simulink model "Part4_solarpanel"  (R2022b)
settings: Solver=FixedStepAuto  StartTime=0.0  StopTime=20  FixedStep=0.0001  RelTol=1e-3
libraries: fl_lib x8, nesl_utility x8, ee_lib x2, simulink x2
settings Model: Creator=mingreico  LastModifiedBy=mingreico

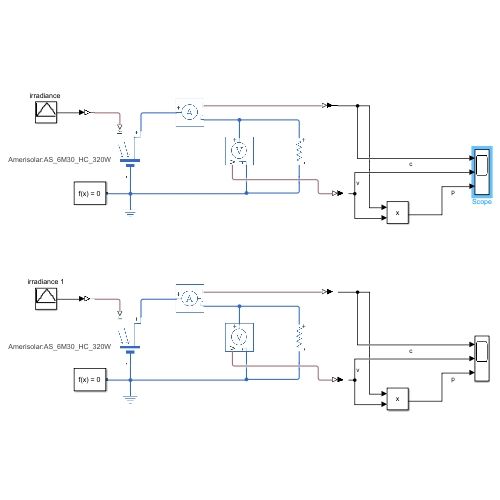
[thumbnail: Simulink's stored preview of the top-level diagram]
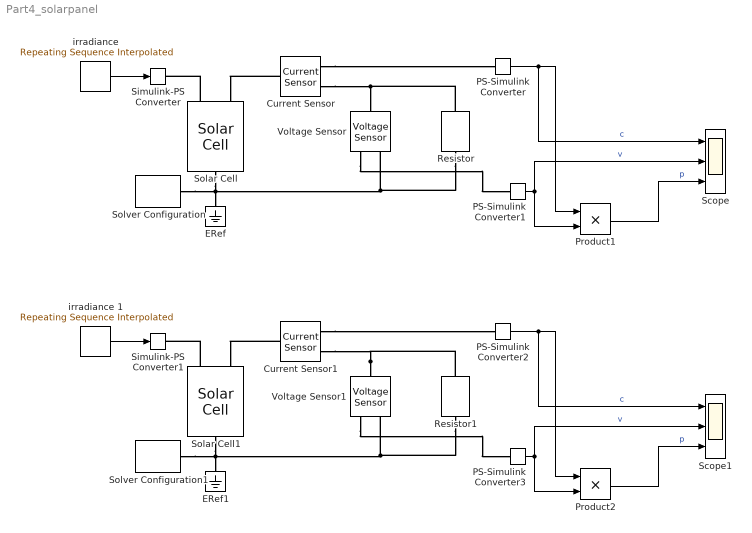
== system Part4_solarpanel ==
  Current Sensor : fl_lib/Electrical/Electrical Sensors/Current Sensor
  Current Sensor1 : fl_lib/Electrical/Electrical Sensors/Current Sensor
  ERef : fl_lib/Electrical/Electrical Elements/Electrical Reference
  ERef1 : fl_lib/Electrical/Electrical Elements/Electrical Reference
  PS-Simulink Converter{,1..3} (4 alike) : nesl_utility/PS-Simulink Converter  PhysicalDomain=network_engine_domain  SubClassName=ps_output  LeftPortType=input  RightPortType=output  PseudoPeriodic=off  Frequencies=[]  VectorFormat=inherit  Unit=inherit  AffineConversion=off
  Product1 : Product
  Product2 : Product
  Resistor : fl_lib/Electrical/Electrical Elements/Resistor  R=100 Ohm  i_specify=off  i_priority=None  i=0 A  i_nominal_specify=off  i_nominal_unit=A  i_nominal_value=1  v_specify=off  v_priority=None  v=0 V  v_nominal_specify=off  v_nominal_unit=V  v_nominal_value=1
  Resistor1 : fl_lib/Electrical/Electrical Elements/Resistor  R=100 Ohm  i_specify=off  i_priority=None  i=0 A  i_nominal_specify=off  i_nominal_unit=A  i_nominal_value=1  v_specify=off  v_priority=None  v=0 V  v_nominal_specify=off  v_nominal_unit=V  v_nominal_value=1
  Scope : Scope  NumInputPorts=3
  Scope1 : Scope  NumInputPorts=3
  Simulink-PS Converter : nesl_utility/Simulink-PS Converter  PhysicalDomain=network_engine_domain  SubClassName=ps_input  LeftPortType=input  RightPortType=output  PseudoPeriodic=off  Frequencies=[]  NoiseDistribution=none  NoiseParameters=[]  Unit=1  AffineConversion=off  FilteringAndDerivatives=provide  SimscapeFilterOrder=1  InputFilterTimeConstant=0.001  UdotUserProvided=0
  Simulink-PS Converter1 : nesl_utility/Simulink-PS Converter  PhysicalDomain=network_engine_domain  SubClassName=ps_input  LeftPortType=input  RightPortType=output  PseudoPeriodic=off  Frequencies=[]  NoiseDistribution=none  NoiseParameters=[]  Unit=1  AffineConversion=off  FilteringAndDerivatives=provide  SimscapeFilterOrder=1  InputFilterTimeConstant=0.001  UdotUserProvided=0
  Solar Cell : ee_lib/Sources/Solar Cell  Tag={'toolbox/physmod/elec/library/m/ee_lib_parts';'Sources/Solar_Cell/Amerisolar/AS_6M30_HC_320W.xml'}  prm=3  Isc=10.14 A  Voc=0.67 V  Is=3.24823447983853e-07 A  Is2=9.37081970792037e-10 A  Iph=10.140005507508 A  Ir0=1000 W/m^2  ec=1.51118472243322  N2=2.60259908345858  Rs=1.94548269975201e-05 Ohm  Rp=682.95993142779 Ohm  N_series=600  N_parallel=1  TIPH1=0.000499942933005141 1/K  EG=1.12 eV  TXIS1=4.23641510120988  TXIS2=16.2689137700667  TRS1=0.243341028305912  TRP1=0 % Parameter not set  Tmeas=25 degC  TFIXED=30 degC  thermal_mass=100 % Parameter not set J/K  initial_temperature=25 degC
      settings: AttributesFormatString=Amerisolar:AS_6M30_HC_320W
  Solar Cell1 : ee_lib/Sources/Solar Cell  Tag={'toolbox/physmod/elec/library/m/ee_lib_parts';'Sources/Solar_Cell/Amerisolar/AS_6M30_HC_320W.xml'}  prm=3  Isc=10.14 A  Voc=0.67 V  Is=3.24823447983853e-07 A  Is2=9.37081970792037e-10 A  Iph=10.140005507508 A  Ir0=1000 W/m^2  ec=1.51118472243322  N2=2.60259908345858  Rs=1.94548269975201e-05 Ohm  Rp=682.95993142779 Ohm  N_series=60  N_parallel=1  TIPH1=0.000499942933005141 1/K  EG=1.12 eV  TXIS1=4.23641510120988  TXIS2=16.2689137700667  TRS1=0.243341028305912  TRP1=0 % Parameter not set  Tmeas=25 degC  TFIXED=25 degC  thermal_mass=100 % Parameter not set J/K  initial_temperature=25 degC
      settings: AttributesFormatString=Amerisolar:AS_6M30_HC_320W
  Solver Configuration : nesl_utility/Solver Configuration  PhysicalDomain=network_engine_domain  SubClassName=solver  LeftPortType=input  RightPortType=generic  Tones=[]  Harmonics=[]  SimulateNoise=off  Profile=off  UseLocalSampling=off  EnableSwitchedLinearOptims=on  FrequencyDomain=off  UseCCode=off  RelTol=0.001  AbsTol=0.001  MinStep=1e-09  ToWorkspace=off  RevertToSquareIcSolve=off  NumHomotopyIterations=100  PhasorMode=off  PhasorModeNumHarmonics=1  ConsistencySolver=NEWTON_XTOL_AFTER_FTOL  IndexReductionMethod=DerivativeReplacement  DoDC=off  ResidualTolerance=1e-09  ConsistencyTolSource=GLOBAL  ConsistencyAbsTol=0.001  ConsistencyRelTol=0.001  ConsistencyTolFactor=0.001  UseLocalSolver=off  LocalSolverChoice=NE_BACKWARD_EULER_ADVANCER  ResolveIndetEquations=on  FunctionEvalNumThread=1  LocalSolverSampleTime=0.001  DoFixedCost=off  MaxNonlinIter=3  MaxModeIter=2  ComputeImpulses=off  ImpulseIterations=2  LinearAlgebra=auto  LinearAlgebraNumThread=0  EquationFormulation=NE_TIME_EF  DelaysMemoryBudget=1024  AutomaticFiltering=on  FilteringTimeConstant=0.0001  PartitionStorageMethod=AS_NEEDED  PartitionMemoryBudget=1024  PartitionMethod=ROBUST
  Solver Configuration1 : nesl_utility/Solver Configuration  PhysicalDomain=network_engine_domain  SubClassName=solver  LeftPortType=input  RightPortType=generic  Tones=[]  Harmonics=[]  SimulateNoise=off  Profile=off  UseLocalSampling=off  EnableSwitchedLinearOptims=on  FrequencyDomain=off  UseCCode=off  RelTol=0.001  AbsTol=0.001  MinStep=1e-09  ToWorkspace=off  RevertToSquareIcSolve=off  NumHomotopyIterations=100  PhasorMode=off  PhasorModeNumHarmonics=1  ConsistencySolver=NEWTON_XTOL_AFTER_FTOL  IndexReductionMethod=DerivativeReplacement  DoDC=off  ResidualTolerance=1e-09  ConsistencyTolSource=GLOBAL  ConsistencyAbsTol=0.001  ConsistencyRelTol=0.001  ConsistencyTolFactor=0.001  UseLocalSolver=off  LocalSolverChoice=NE_BACKWARD_EULER_ADVANCER  ResolveIndetEquations=on  FunctionEvalNumThread=1  LocalSolverSampleTime=0.001  DoFixedCost=off  MaxNonlinIter=3  MaxModeIter=2  ComputeImpulses=off  ImpulseIterations=2  LinearAlgebra=auto  LinearAlgebraNumThread=0  EquationFormulation=NE_TIME_EF  DelaysMemoryBudget=1024  AutomaticFiltering=on  FilteringTimeConstant=0.0001  PartitionStorageMethod=AS_NEEDED  PartitionMemoryBudget=1024  PartitionMethod=ROBUST
  Voltage Sensor : fl_lib/Electrical/Electrical Sensors/Voltage Sensor
  Voltage Sensor1 : fl_lib/Electrical/Electrical Sensors/Voltage Sensor
  "irradiance " : simulink/Sources/Repeating Sequence Interpolated  OutValues=[0 0 1 1 2 2 3 3 4 4 5 5 6 6 5 5 4 4 3 3 2 2 1 1]*200  TimeValues=[0 1 2 3 4 5 6 7 8 9 10 11 12 13 14 15 16 17 18 19 20 21 22 23]  LookUpMeth=Interpolation-Use End Values  tsamp=1e-4  OutMin=[]  OutMax=[]  OutDataTypeStr=double  OutputDataTypeScalingMode=double  OutDataType=fixdt(0,8)  OutScaling=2^-10
  irradiance 1 : simulink/Sources/Repeating Sequence Interpolated  OutValues=[0 0 1 1 2 2 3 3 4 4 5 5 6 6 5 5 4 4 3 3 2 2 1 1]*200  TimeValues=[0 1 2 3 4 5 6 7 8 9 10 11 12 13 14 15 16 17 18 19 20 21 22 23]  LookUpMeth=Interpolation-Use End Values  tsamp=1e-4  OutMin=[]  OutMax=[]  OutDataTypeStr=double  OutputDataTypeScalingMode=double  OutDataType=fixdt(0,8)  OutScaling=2^-10
  wires:
  "irradiance "/1 -> Simulink-PS Converter/1
  PS-Simulink Converter/1 -> Product1/1, Scope/1  "c"
  PS-Simulink Converter1/1 -> Product1/2, Scope/2  "v"
  Product1/1 -> Scope/3  "p"
  PS-Simulink Converter3/1 -> Product2/2, Scope1/2  "v"
  PS-Simulink Converter2/1 -> Product2/1, Scope1/1  "c"
  irradiance 1/1 -> Simulink-PS Converter1/1
  Product2/1 -> Scope1/3  "p"
  connections:
  Solar Cell/RConn1 -- Resistor/RConn1 -- Voltage Sensor/RConn2 -- Solver Configuration/RConn1 -- ERef/LConn1
  Current Sensor/LConn1 -- Solar Cell/LConn2
  Solar Cell/LConn1 -- Simulink-PS Converter/RConn1
  Current Sensor/RConn2 -- Resistor/LConn1 -- Voltage Sensor/LConn1
  Current Sensor/RConn1 -- PS-Simulink Converter/LConn1
  Voltage Sensor/RConn1 -- PS-Simulink Converter1/LConn1
  Voltage Sensor1/LConn1 -- Current Sensor1/RConn2 -- Resistor1/LConn1
  Solar Cell1/RConn1 -- Resistor1/RConn1 -- Voltage Sensor1/RConn2 -- Solver Configuration1/RConn1 -- ERef1/LConn1
  Solar Cell1/LConn1 -- Simulink-PS Converter1/RConn1
  Voltage Sensor1/RConn1 -- PS-Simulink Converter3/LConn1
  Current Sensor1/RConn1 -- PS-Simulink Converter2/LConn1
  Current Sensor1/LConn1 -- Solar Cell1/LConn2
